simulink model "dc_pidmotor"  (Simulink 10.1)
settings: Solver=ode45  StartTime=0.0  StopTime=50  RelTol=1e-3  EnableMultiTasking=on
libraries: simulink x1
settings Model: Creator=lenovo  LastModifiedBy=blaze8871
settings DataIOCC: LimitDataPoints=on  SignalLoggingSaveFormat=ModelDataLogs
settings OptimizationCC: ExpressionDepthLimit=2147483647
settings DebuggingCC: SolverPrmCheckMsg=warning  FcnCallInpInsideContextMsg=warning  StateNameClashWarn=warning  SFExecutionAtInitializationDiag=warning
settings GRTTargetCC: CombineOutputUpdateFcns=on  GRTInterface=off

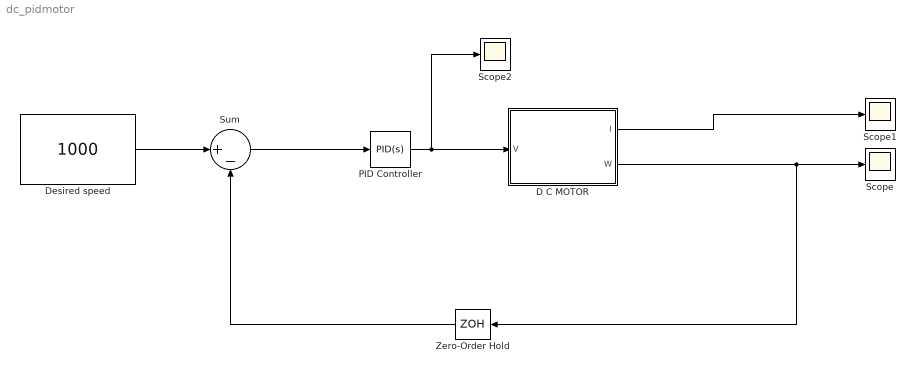
== system dc_pidmotor ==
  D C MOTOR : Subsystem
  Desired speed : Constant  Value=1000
  PID Controller : simulink/Continuous/PID Controller  Controller=PID  Form=Parallel  TimeDomain=Continuous-time  UseExternalTs=off  SampleTime=-1  IntegratorMethod=Forward Euler  FilterMethod=Forward Euler  ControllerParametersSource=internal  P=0.507985839103074  I=0.16898150885466  D=-0.183693228810871  UseFilter=on  N=2.16794558670696  TunerSelectOption=Transfer Function Based (PID Tuner App)  InitialConditionSource=internal  InitialConditionForIntegrator=0  InitialConditionForFilter=0  DifferentiatorICPrevScaledInput=0  ExternalReset=none  TrackingMode=off  Kt=1  LimitOutput=off  UpperSaturationLimit=inf  LowerSaturationLimit=-inf  LinearizeAsGain=on  AntiWindupMode=none  Kb=1  POutMin=[]  POutMax=[]  IOutMin=[]  IOutMax=[]  DOutMin=[]  DOutMax=[]  NOutMin=[]  NOutMax=[]  SumOutMin=[]  SumOutMax=[]  SaturationOutMin=[]  SaturationOutMax=[]  PParamMin=[]  PParamMax=[]  IParamMin=[]  IParamMax=[]  DParamMin=[]  DParamMax=[]  NParamMin=[]  NParamMax=[]  KbParamMin=[]  KbParamMax=[]  KtParamMin=[]  KtParamMax=[]  KbOutMin=[]  KbOutMax=[]  KtOutMin=[]  KtOutMax=[]  IntegratorOutMin=[]  IntegratorOutMax=[]  FilterOutMin=[]  FilterOutMax=[]  SumI1OutMin=[]  SumI1OutMax=[]  SumI2OutMin=[]  SumI2OutMax=[]  SumI3OutMin=[]  SumI3OutMax=[]  SumI4OutMin=[]  SumI4OutMax=[]  SumDOutMin=[]  SumDOutMax=[]  DifferentiatorOutMin=[]  DifferentiatorOutMax=[]  FilterDiffOutCoefMin=[]  FilterDiffOutCoefMax=[]  ReciprocalOutMin=[]  ReciprocalOutMax=[]  SumDenOutMin=[]  SumDenOutMax=[]  SumNumOutMin=[]  SumNumOutMax=[]  DivideOutMin=[]  DivideOutMax=[]  UdiffTsProdOutMin=[]  UdiffTsProdOutMax=[]  NTsProdOutMin=[]  NTsProdOutMax=[]  UintegralTsProdOutMin=[]  UintegralTsProdOutMax=[]  UngainTsProdOutMin=[]  UngainTsProdOutMax=[]  IntegratorContinuousStateAttributes=''  IntegratorStateMustResolveToSignalObject=off  IntegratorRTWStateStorageClass=Auto  FilterContinuousStateAttributes=''  FilterStateMustResolveToSignalObject=off  FilterRTWStateStorageClass=Auto  ParallelPVariant=InternalParameters  IdealPVariant=Disabled  IVariant=InternalParameters  DVariant=InternalParameters  IntegratorVariant=Continuous  SatVariant=Disabled  AWVariant=Passthrough  PCopyVariant=Disabled  TRVariant=Disabled  FdbkBlocksVariant=Forward  IdealPFdbkVariant=Disabled  SatFdbkVariant=Disabled  DerivativeFilterVariant=ContFilter  NVariant=InternalParameters  NCopyVariant=Disabled  FilterICVariant=InternalICsFilter  IntegratorICVariant=InternalICs  ExternalResetVariant=Disabled  TRSumVariant=Passthrough  SumFdbkVariant=Disabled  SumVariant=Sum_PID  TsampFilterVariant=InternalTs  TsampNgainVariant=Passthrough  TsampIntegralVariant=Passthrough
  Scope : Scope
  Scope1 : Scope
  Scope2 : Scope
  Sum : Sum  Inputs=|+-
  Zero-Order Hold : ZeroOrderHold
  wires:
  D C MOTOR/1(I) -> Scope1/1
  Desired speed/1 -> Sum/1
  D C MOTOR/2(W) -> Zero-Order Hold/1, Scope/1
  Zero-Order Hold/1 -> Sum/2
  Sum/1 -> PID Controller/1
  PID Controller/1 -> Scope2/1, D C MOTOR/1(V)

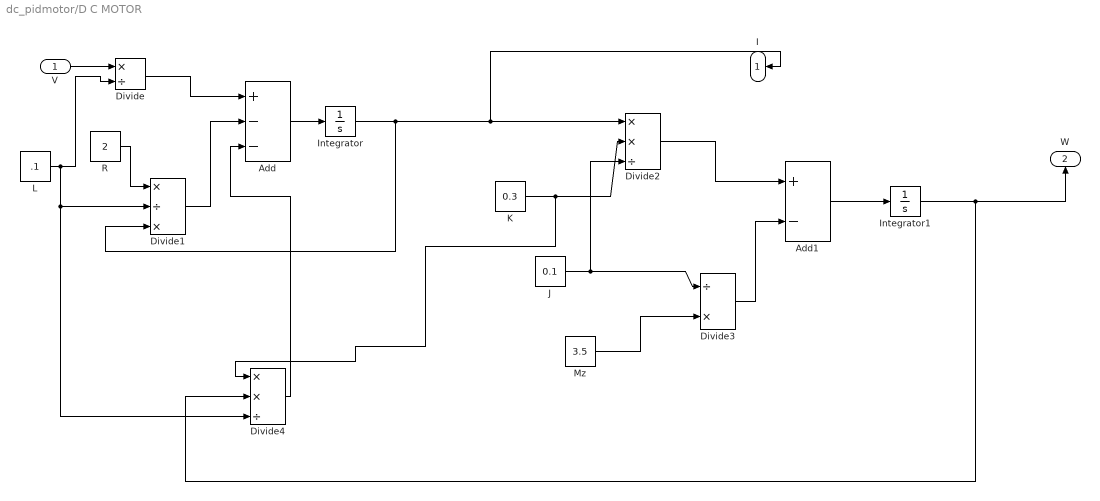
== system dc_pidmotor/D C MOTOR ==
  V : Inport
  Add : Sum  Inputs=+--
  Add1 : Sum  Inputs=+-
  Divide : Product  Inputs=*/
  Divide1 : Product  Inputs=*/*
  Divide2 : Product  Inputs=**/
  Divide3 : Product  Inputs=/*
  Divide4 : Product  Inputs=**/
  Integrator : Integrator
  Integrator1 : Integrator
  J : Constant  Value=0.1
  K : Constant  Value=0.3
  L : Constant  Value=.1
  Mz : Constant  Value=3.5
  R : Constant  Value=2
  I : Outport
  W : Outport  Port=2
  wires:
  L/1 -> Divide/2, Divide1/2, Divide4/3
  Add/1 -> Integrator/1
  Divide/1 -> Add/1
  R/1 -> Divide1/1
  Integrator/1 -> Divide1/3, Divide2/1, I/1
  K/1 -> Divide2/2, Divide4/1
  J/1 -> Divide2/3, Divide3/1
  Divide2/1 -> Add1/1
  Mz/1 -> Divide3/2
  Divide3/1 -> Add1/2
  Add1/1 -> Integrator1/1
  Divide1/1 -> Add/2
  Divide4/1 -> Add/3
  Integrator1/1 -> Divide4/2, W/1
  V/1 -> Divide/1
